simulink model "Model3"  (R2020a)
settings: Solver=VariableStepAuto  StartTime=0.0  StopTime=16*(1.302083333333333e-07)  RelTol=1e-3
undefined symbols (not defined in the file or in its folder): pskmod
libraries: commdigbbndpm3 x2, commutil2 x2, commrandsrc3 x1, commsink2 x1
settings Model: Creator=esha_  LastModifiedBy=esha_

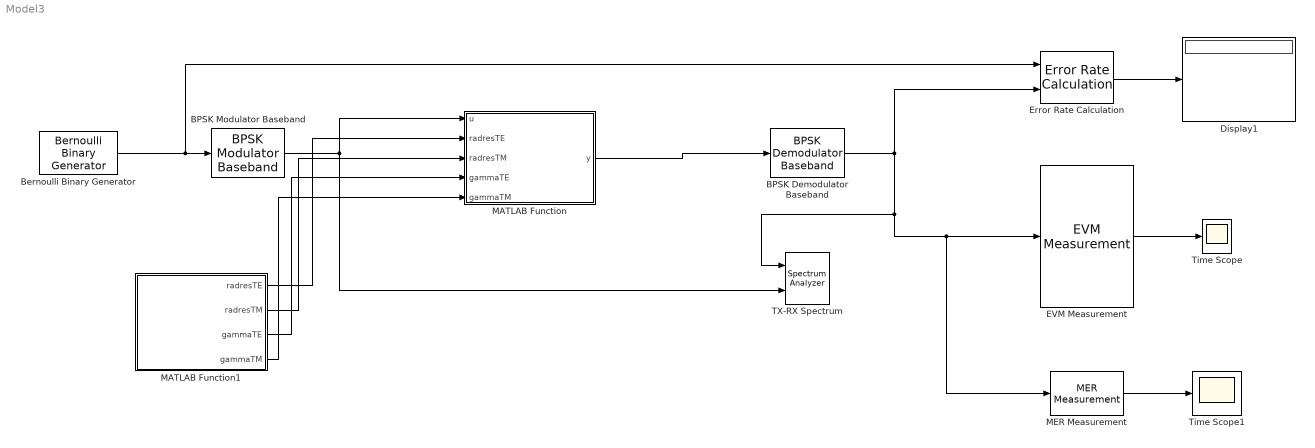
== system Model3 ==
  BPSK Demodulator Baseband : commdigbbndpm3/BPSK Demodulator Baseband  DecType=Hard decision  VarSource=Dialog  Variance=1  Ph=0  outDtype=Inherit via internal rule  derotateFactorWordLen=16  derotateFactorDataTypeStr=Inherit: Same word length as input  derotateFactorLastDataTypeStr=Inherit: Same word length as input
  BPSK Modulator Baseband : commdigbbndpm3/BPSK Modulator Baseband  Ph=0  outDtype=double  outWordLen=16  outUDDataType=sfix(16)  outFracLenMode=Best precision  outFracLen=15  outDataTypeStr=double  outLastDataTypeStr=double
  Bernoulli Binary Generator : commrandsrc3/Bernoulli Binary Generator  ProbabilityOfZero=0.5  SeedSource=Parameter  Seed=61  SampleTime=1.302083333333333e-07  SamplesPerFrame=5000  OutputDataType=double  SimulateUsing=Code generation
  Display1 : Display
  EVM Measurement : commutil2/EVM Measurement  Normalization=Average reference signal power  AverageConstellationPower=1  PeakConstellationPower=1  ReferenceSignalSource=Estimated from reference constellation  ReferenceConstellation=pskmod((0:1),2,0)  MeasurementIntervalSource=Input length  MeasurementInterval=100  AveragingDimensions=1  MaximumEVMOutputPort=off  XPercentileEVMOutputPort=off  XPercentileValue=95  SymbolCountOutputPort=on  SimulateUsing=Interpreted execution
      settings: SourceProductBaseCode=CM
  Error Rate Calculation : commsink2/Error Rate Calculation  N=0  st_delay=0  cp_mode=Entire frame  subframe=[]  PMode=Port  WsName=ErrorVec  RsMode2=off  stop=on  numErr=100  maxBits=1e6
  MATLAB Function : MATLAB Function  TreatAsAtomicUnit=on
  MATLAB Function1 : MATLAB Function  TreatAsAtomicUnit=on
  MER Measurement : commutil2/MER Measurement  ReferenceSignalSource=Estimated from reference constellation  ReferenceConstellation=pskmod((0:1),2,0)  MeasurementIntervalSource=Input length  MeasurementInterval=100  AveragingDimensions=1  MinimumMEROutputPort=off  XPercentileMEROutputPort=off  XPercentileValue=95  SymbolCountOutputPort=off  SimulateUsing=Interpreted execution
      settings: SourceProductBaseCode=CM
  TX-RX Spectrum : SpectrumAnalyzer  NumInputPorts=2
  Time Scope : Scope
      settings: Description=EVM
  Time Scope1 : Scope
      settings: Description=SNR
  wires:
  BPSK Demodulator Baseband/1 -> MER Measurement/1, EVM Measurement/1, TX-RX Spectrum/1, Error Rate Calculation/2
  BPSK Modulator Baseband/1 -> MATLAB Function/1(u), TX-RX Spectrum/2
  EVM Measurement/1 -> Time Scope/1
  Error Rate Calculation/1 -> Display1/1
  MER Measurement/1 -> Time Scope1/1
  Bernoulli Binary Generator/1 -> Error Rate Calculation/1, BPSK Modulator Baseband/1
  MATLAB Function/1(y) -> BPSK Demodulator Baseband/1
  MATLAB Function1/1(radresTE) -> MATLAB Function/2(radresTE)
  MATLAB Function1/2(radresTM) -> MATLAB Function/3(radresTM)
  MATLAB Function1/3(gammaTE) -> MATLAB Function/4(gammaTE)
  MATLAB Function1/4(gammaTM) -> MATLAB Function/5(gammaTM)

== matlab function Model3/MATLAB Function1 ==
  data: radresTE output; radresTM output; gammaTE output; gammaTM output
function [radresTE, radresTM, gammaTE, gammaTM] = fcn()
radresTE1 = load('radresTE.mat');
radresTE = radresTE1.radresTE;
radresTM1 = load('radresTM.mat');
radresTM = radresTM1.radresTM;
gammaTE1 = load('gammaTE.mat');
gammaTE = gammaTE1.gammaTE;
gammaTM1 = load('gammaTM.mat');
gammaTM = gammaTM1.gammaTM;
end

== matlab function Model3/MATLAB Function ==
  data: y output; u input; radresTE input; radresTM input; gammaTE input; gammaTM input
function y = fcn(u,radresTE, radresTM, gammaTE, gammaTM)
freq = 59E9:4E6:60E9; 
n_TE = 0;
n_TM = 17;
Zo=50;
WGlen = 5;

radreacTE = imag(hilbert(radresTE));
radreacTM = imag(hilbert(radresTM));
antresTE = zeros(1,length(freq));
antresTM = zeros(1,length(freq));
antreacTE = zeros(1,length(freq));
antreacTM = zeros(1,length(freq));
antimpTE = zeros(1,length(freq)) + 1i*zeros(1,length(freq));
antimpTM = zeros(1,length(freq)) + 1i*zeros(1,length(freq));
TEmodeimp = zeros(length(freq), length(n_TE)) + 1i*zeros(length(freq), length(n_TE));
TMmodeimp = zeros(length(freq), length(n_TM)) + 1i*zeros(length(freq), length(n_TM));
channel = zeros(1,length(freq)) + 1i*zeros(1,length(freq));
for fi=1:length(freq)
    antresTE(fi) = sum(radresTE(fi,:));
    antresTM(fi) = sum(radresTM(fi,:));
    antreacTE(fi) = sum(radreacTE(fi,:));
    antreacTM(fi) = sum(radreacTM(fi,:));
    antimpTE(fi) = antresTE(fi) +1i*antreacTE(fi);
    antimpTM(fi) = antresTM(fi) +1i*antreacTM(fi);
    for n = 1:length(n_TE)
        TEmodeimp(fi,n)=radresTE(fi,n)+1i*radreacTE(fi,n);
    end
    for n = 1:length(n_TM)
        TMmodeimp(fi,n)=radresTM(fi,n)+1i*radreacTM(fi,n);
    end    
end
for fi=1:length(freq)
    %TsTE = diag(exp(-1*gammaTE(fi,:)*WGlen));
    %chTEmode = TEmodeimp(fi,:)*TsTE;
    TsTM = diag(exp(-1*gammaTM(fi,:)*WGlen));
    chTMmode = TMmodeimp(fi,:)*TsTM;
    channel(fi) = ((2*Zo)/(abs(Zo + antimpTM(fi))^2))*...
        (sum(chTMmode));
%     channel(fi) = ((2*Zo)/(abs(antimpTM(fi) + Zo + antimpTE(fi))^2))*...
%         (sum(chTEmode)+sum(chTMmode));
end
% uu = u';
% cchanel = channel';
y = conv(u,channel,'same');
%y = channel;
